simulink model "dual_single_phase_parallel_inverter_r2024a"  (R2024a)
settings: Solver=ode23t  StartTime=0.0  StopTime=0.25  MaxStep=5e-6  RelTol=1e-4
model workspace (MAT data in the model file):
  Paux1_W = 1
  Paux2_W = 1
libraries: nesl_utility x41, fl_lib x39, ee_lib x31, simulink x6
(part 1 of 4)
settings Model: Creator=chidan  LastModifiedBy=chidan

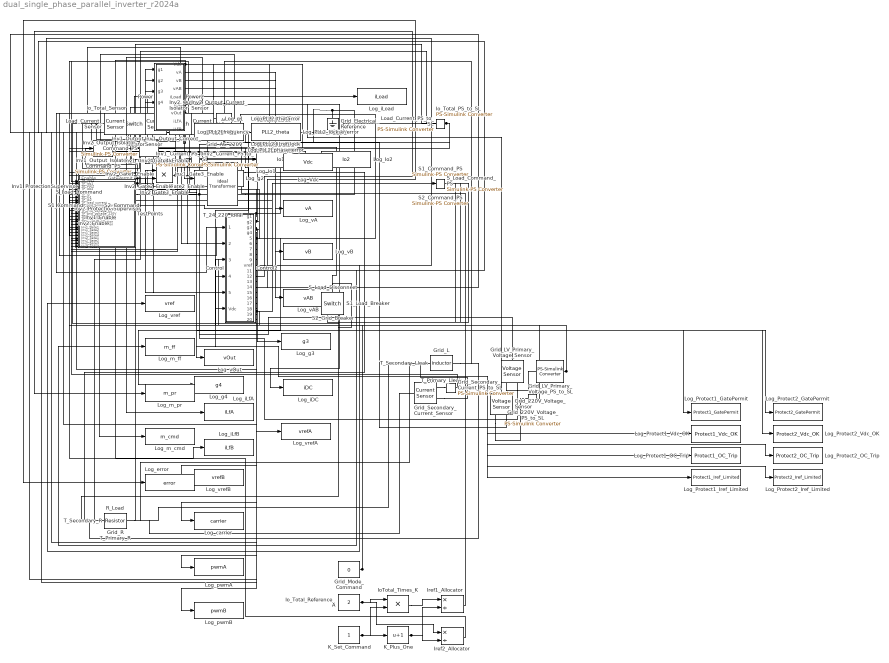
== system dual_single_phase_parallel_inverter_r2024a ==
  Control : Subsystem
  Control2 : Subsystem
  Grid_220V_Voltage_PS_to_SL : nesl_utility/PS-Simulink Converter  PhysicalDomain=network_engine_domain  SubClassName=ps_output  LeftPortType=input  RightPortType=output  PseudoPeriodic=off  Frequencies=[]  VectorFormat=inherit  Unit=inherit  AffineConversion=off
  Grid_220V_Voltage_Sensor : fl_lib/Electrical/Electrical Sensors/Voltage Sensor
  Grid_AC_220V : fl_lib/Electrical/Electrical Sources/AC Voltage Source  amp=220*sqrt(2) V  shift=0 rad  frequency=50 Hz
  Grid_Electrical_Reference : fl_lib/Electrical/Electrical Elements/Electrical Reference
  Grid_L : ee_lib/Passive/Inductor  l=1e-3 H  enable_L_tol=ee.enum.toleranceApplication.none  L_tol=20  tol_distribution=ee.enum.toleranceDistribution.uniform  nSigma=4  r=0.1 Ohm  g=1e-9 1/Ohm  enable_operating_limits=ee.enum.enable.no  operating_limit_action=ee.enum.passive.reportOpLim.warn  max_working_current=1 A  power_rating=1 W  enable_faults=ee.enum.enable.no  fault_action=simscape.enum.assert.action.none  lambdaPercent=50  k_faulted=0.9999  turnsShort=ee.enum.passive.inductor.turnsShortOption.no  openCct=ee.enum.enable.no  groundShort=ee.enum.passive.inductor.groundShortOption.no  groundShortG=0 1/Ohm  tau_fault=1e-3 s  fault_trigger=ee.enum.faults.faultTrigger.temporal  t_fault=1 s  max_permissible_voltage=100 V  n_fail_on_voltage=1  max_permissible_current=1 A  t_fail_on_current=1 s  i_L_specify=off  i_L_priority=High  i_L=0 A  i_L_nominal_specify=off  i_L_nominal_value=1  i_L_nominal_unit=A  faulted_specify=off  faulted_priority=None  faulted=0
  Grid_LV_Primary_Voltage_PS_to_SL : nesl_utility/PS-Simulink Converter  PhysicalDomain=network_engine_domain  SubClassName=ps_output  LeftPortType=input  RightPortType=output  PseudoPeriodic=off  Frequencies=[]  VectorFormat=inherit  Unit=inherit  AffineConversion=off
  Grid_LV_Primary_Voltage_Sensor : fl_lib/Electrical/Electrical Sensors/Voltage Sensor
  Grid_Mode_Command : Constant  Value=0
  Grid_R : ee_lib/Passive/Resistor  R=0.5 Ohm  enable_R_tol=ee.enum.toleranceApplication.none  R_tol=5  tol_distribution=ee.enum.toleranceDistribution.uniform  nSigma=4  enable_operating_limits=ee.enum.enable.no  operating_limit_action=ee.enum.passive.reportOpLim.warn  power_rating=1 W  max_working_voltage=100 V  enable_faults=ee.enum.enable.no  fault_action=simscape.enum.assert.action.none  R_faulted=inf Ohm  fault_trigger=ee.enum.faults.faultTrigger.temporal  t_fault=1 s  max_permissible_current=1 A  t_fail_on_current=1 s  noise_mode=ee.enum.sources.noise.Disabled  Tdevice=25 degC  sample_time=1e-3 s  repeatability=ee.enum.ic.repeatability.notRepeatable  user_seed=0  auto_seed=2348838240  faulted_specify=off  faulted_priority=None  faulted=0  power_derating_T1=70 degC  power_derating_T2=155 degC  operating_temperature_range_vec=[-50, 150] degC  alpha=3.93e-3 1/K  Tmeas=25 degC  thermal_mass=100 J/K  temperature_specify=off  temperature_priority=High  temperature=298.15 K  temperature_nominal_specify=off  temperature_nominal_value=1  temperature_nominal_unit=K
  Grid_Secondary_Current_PS_to_SL : nesl_utility/PS-Simulink Converter  PhysicalDomain=network_engine_domain  SubClassName=ps_output  LeftPortType=input  RightPortType=output  PseudoPeriodic=off  Frequencies=[]  VectorFormat=inherit  Unit=inherit  AffineConversion=off
  Grid_Secondary_Current_Sensor : fl_lib/Electrical/Electrical Sensors/Current Sensor
  Inv1_Current_PS_to_SL : nesl_utility/PS-Simulink Converter  PhysicalDomain=network_engine_domain  SubClassName=ps_output  LeftPortType=input  RightPortType=output  PseudoPeriodic=off  Frequencies=[]  VectorFormat=inherit  Unit=inherit  AffineConversion=off
  Inv1_Enable : Constant
  Inv1_Gate1_Enable : Product
  Inv1_Gate2_Enable : Product
  Inv1_Gate3_Enable : Product
  Inv1_Gate4_Enable : Product
  Inv1_Output_Current_Sensor : fl_lib/Electrical/Electrical Sensors/Current Sensor
  Inv1_Output_Isolator : fl_lib/Electrical/Electrical Elements/Switch  R_closed=0.001 Ohm  G_open=1e-8 1/Ohm  Threshold=0.5  i_specify=off  i_priority=None  i=0 A  i_nominal_specify=off  i_nominal_value=1  i_nominal_unit=A  v_specify=off  v_priority=None  v=0 V  v_nominal_specify=off  v_nominal_value=1  v_nominal_unit=V
  Inv1_Output_Isolator_Command_PS : nesl_utility/Simulink-PS Converter  PhysicalDomain=network_engine_domain  SubClassName=ps_input  LeftPortType=input  RightPortType=output  PseudoPeriodic=off  Frequencies=[]  NoiseDistribution=none  NoiseParameters=[]  Unit=1  AffineConversion=off  FilteringAndDerivatives=provide  SimscapeFilterOrder=1  InputFilterTimeConstant=0.001  UdotUserProvided=0
  Inv1_ProtectionSupervisor : Subsystem
  Inv2_Current_PS_to_SL : nesl_utility/PS-Simulink Converter  PhysicalDomain=network_engine_domain  SubClassName=ps_output  LeftPortType=input  RightPortType=output  PseudoPeriodic=off  Frequencies=[]  VectorFormat=inherit  Unit=inherit  AffineConversion=off
  Inv2_Enable : Constant
  Inv2_Gate1_Enable : Product
  Inv2_Gate2_Enable : Product
  Inv2_Gate3_Enable : Product
  Inv2_Gate4_Enable : Product
  Inv2_Output_Current_Sensor : fl_lib/Electrical/Electrical Sensors/Current Sensor
  Inv2_Output_Isolator : fl_lib/Electrical/Electrical Elements/Switch  R_closed=0.001 Ohm  G_open=1e-8 1/Ohm  Threshold=0.5  i_specify=off  i_priority=None  i=0 A  i_nominal_specify=off  i_nominal_value=1  i_nominal_unit=A  v_specify=off  v_priority=None  v=0 V  v_nominal_specify=off  v_nominal_value=1  v_nominal_unit=V
  Inv2_Output_Isolator_Command_PS : nesl_utility/Simulink-PS Converter  PhysicalDomain=network_engine_domain  SubClassName=ps_input  LeftPortType=input  RightPortType=output  PseudoPeriodic=off  Frequencies=[]  NoiseDistribution=none  NoiseParameters=[]  Unit=1  AffineConversion=off  FilteringAndDerivatives=provide  SimscapeFilterOrder=1  InputFilterTimeConstant=0.001  UdotUserProvided=0
  Inv2_ProtectionSupervisor : Subsystem
  IoTotal_Times_K : Product  Inputs=**
  Io_Total_PS_to_SL : nesl_utility/PS-Simulink Converter  PhysicalDomain=network_engine_domain  SubClassName=ps_output  LeftPortType=input  RightPortType=output  PseudoPeriodic=off  Frequencies=[]  VectorFormat=inherit  Unit=inherit  AffineConversion=off
  Io_Total_Reference_A : Constant  Value=2
  Io_Total_Sensor : fl_lib/Electrical/Electrical Sensors/Current Sensor
  Iref1_Allocator : Product  Inputs=*/
  Iref2_Allocator : Product  Inputs=*/
  K_Plus_One : Bias  Bias=1  SaturateOnIntegerOverflow=off
  K_Set_Command : Constant
  Load_Current_PS_to_SL : nesl_utility/PS-Simulink Converter  PhysicalDomain=network_engine_domain  SubClassName=ps_output  LeftPortType=input  RightPortType=output  PseudoPeriodic=off  Frequencies=[]  VectorFormat=inherit  Unit=inherit  AffineConversion=off
  Load_Current_Sensor : fl_lib/Electrical/Electrical Sensors/Current Sensor
  Log_Inv1_Gate1 : ToWorkspace  VariableName=Inv1_gate1  SaveFormat=Timeseries  SampleTime=-1
  Log_Inv1_Gate2 : ToWorkspace  VariableName=Inv1_gate2  SaveFormat=Timeseries  SampleTime=-1
  Log_Inv1_Gate3 : ToWorkspace  VariableName=Inv1_gate3  SaveFormat=Timeseries  SampleTime=-1
  Log_Inv1_Gate4 : ToWorkspace  VariableName=Inv1_gate4  SaveFormat=Timeseries  SampleTime=-1
  Log_Inv2_Ctrl_g1 : ToWorkspace  VariableName=Inv2_ctrl_g1  SaveFormat=Timeseries  SampleTime=-1
  Log_Inv2_Ctrl_g2 : ToWorkspace  VariableName=Inv2_ctrl_g2  SaveFormat=Timeseries  SampleTime=-1
  Log_Inv2_Ctrl_g3 : ToWorkspace  VariableName=Inv2_ctrl_g3  SaveFormat=Timeseries  SampleTime=-1
  Log_Inv2_Ctrl_g4 : ToWorkspace  VariableName=Inv2_ctrl_g4  SaveFormat=Timeseries  SampleTime=-1
  Log_Inv2_Gate1 : ToWorkspace  VariableName=Inv2_gate1  SaveFormat=Timeseries  SampleTime=-1
  Log_Inv2_Gate2 : ToWorkspace  VariableName=Inv2_gate2  SaveFormat=Timeseries  SampleTime=-1
  Log_Inv2_Gate3 : ToWorkspace  VariableName=Inv2_gate3  SaveFormat=Timeseries  SampleTime=-1
  Log_Inv2_Gate4 : ToWorkspace  VariableName=Inv2_gate4  SaveFormat=Timeseries  SampleTime=-1
  Log_Inv2_Vdc : ToWorkspace  VariableName=Inv2_Vdc  SaveFormat=Timeseries  SampleTime=-1
  Log_Inv2_carrier : ToWorkspace  VariableName=Inv2_carrier  SaveFormat=Timeseries  SampleTime=-1
  Log_Inv2_error : ToWorkspace  VariableName=Inv2_error  SaveFormat=Timeseries  SampleTime=-1
  Log_Inv2_iDC : ToWorkspace  VariableName=Inv2_iDC  SaveFormat=Timeseries  SampleTime=-1
  Log_Inv2_iLfA : ToWorkspace  VariableName=Inv2_iLfA  SaveFormat=Timeseries  SampleTime=-1
  Log_Inv2_iLfB : ToWorkspace  VariableName=Inv2_iLfB  SaveFormat=Timeseries  SampleTime=-1
  Log_Inv2_iLoad : ToWorkspace  VariableName=Inv2_iLoad  SaveFormat=Timeseries  SampleTime=-1
  Log_Inv2_m_cmd : ToWorkspace  VariableName=Inv2_m_cmd  SaveFormat=Timeseries  SampleTime=-1
  Log_Inv2_m_ff : ToWorkspace  VariableName=Inv2_m_ff  SaveFormat=Timeseries  SampleTime=-1
  Log_Inv2_m_pr : ToWorkspace  VariableName=Inv2_m_pr  SaveFormat=Timeseries  SampleTime=-1
  Log_Inv2_pwmA : ToWorkspace  VariableName=Inv2_pwmA  SaveFormat=Timeseries  SampleTime=-1
  Log_Inv2_pwmB : ToWorkspace  VariableName=Inv2_pwmB  SaveFormat=Timeseries  SampleTime=-1
  Log_Inv2_vA : ToWorkspace  VariableName=Inv2_vA  SaveFormat=Timeseries  SampleTime=-1
  Log_Inv2_vAB : ToWorkspace  VariableName=Inv2_vAB  SaveFormat=Timeseries  SampleTime=-1
  Log_Inv2_vB : ToWorkspace  VariableName=Inv2_vB  SaveFormat=Timeseries  SampleTime=-1
  Log_Inv2_vOut : ToWorkspace  VariableName=Inv2_vOut  SaveFormat=Timeseries  SampleTime=-1
  Log_Inv2_vref : ToWorkspace  VariableName=Inv2_vref  SaveFormat=Timeseries  SampleTime=-1
  Log_Inv2_vrefA : ToWorkspace  VariableName=Inv2_vrefA  SaveFormat=Timeseries  SampleTime=-1
  Log_Inv2_vrefB : ToWorkspace  VariableName=Inv2_vrefB  SaveFormat=Timeseries  SampleTime=-1
  Log_Io1 : ToWorkspace  VariableName=Io1  SaveFormat=Timeseries  SampleTime=-1
  Log_Io2 : ToWorkspace  VariableName=Io2  SaveFormat=Timeseries  SampleTime=-1
  Log_Io_Total : ToWorkspace  VariableName=Io_total  SaveFormat=Timeseries  SampleTime=-1
  Log_Load_Current : ToWorkspace  VariableName=I_load  SaveFormat=Timeseries  SampleTime=-1
  Log_PLL1_frequency : ToWorkspace  VariableName=PLL1_frequency_Hz  SaveFormat=Timeseries  SampleTime=-1
  Log_PLL1_i_error : ToWorkspace  VariableName=PLL1_i_error_A  SaveFormat=Timeseries  SampleTime=-1
  Log_PLL1_i_ref : ToWorkspace  VariableName=PLL1_i_ref_A  SaveFormat=Timeseries  SampleTime=-1
  Log_PLL1_lock : ToWorkspace  VariableName=PLL1_lock  SaveFormat=Timeseries  SampleTime=-1
  Log_PLL1_phase_error : ToWorkspace  VariableName=PLL1_phase_error  SaveFormat=Timeseries  SampleTime=-1
  Log_PLL1_theta : ToWorkspace  VariableName=PLL1_theta  SaveFormat=Timeseries  SampleTime=-1
  Log_PLL2_frequency : ToWorkspace  VariableName=PLL2_frequency_Hz  SaveFormat=Timeseries  SampleTime=-1
  Log_PLL2_i_error : ToWorkspace  VariableName=PLL2_i_error_A  SaveFormat=Timeseries  SampleTime=-1
  Log_PLL2_i_ref : ToWorkspace  VariableName=PLL2_i_ref_A  SaveFormat=Timeseries  SampleTime=-1
  Log_PLL2_lock : ToWorkspace  VariableName=PLL2_lock  SaveFormat=Timeseries  SampleTime=-1
  Log_PLL2_phase_error : ToWorkspace  VariableName=PLL2_phase_error  SaveFormat=Timeseries  SampleTime=-1
  Log_PLL2_theta : ToWorkspace  VariableName=PLL2_theta  SaveFormat=Timeseries  SampleTime=-1
  Log_Protect1_GatePermit : ToWorkspace  VariableName=Protect1_GatePermit  SaveFormat=Timeseries  SampleTime=-1
  Log_Protect1_Iref_Limited : ToWorkspace  VariableName=Protect1_Iref_Limited  SaveFormat=Timeseries  SampleTime=-1
  Log_Protect1_OC_Trip : ToWorkspace  VariableName=Protect1_OC_Trip  SaveFormat=Timeseries  SampleTime=-1
  Log_Protect1_Vdc_OK : ToWorkspace  VariableName=Protect1_Vdc_OK  SaveFormat=Timeseries  SampleTime=-1
  Log_Protect2_GatePermit : ToWorkspace  VariableName=Protect2_GatePermit  SaveFormat=Timeseries  SampleTime=-1
  Log_Protect2_Iref_Limited : ToWorkspace  VariableName=Protect2_Iref_Limited  SaveFormat=Timeseries  SampleTime=-1
  Log_Protect2_OC_Trip : ToWorkspace  VariableName=Protect2_OC_Trip  SaveFormat=Timeseries  SampleTime=-1
  Log_Protect2_Vdc_OK : ToWorkspace  VariableName=Protect2_Vdc_OK  SaveFormat=Timeseries  SampleTime=-1
  Log_Vdc : ToWorkspace  VariableName=Vdc  SaveFormat=Timeseries  SampleTime=-1
  Log_carrier : ToWorkspace  VariableName=carrier  SaveFormat=Timeseries  SampleTime=-1
  Log_error : ToWorkspace  VariableName=error  SaveFormat=Timeseries  SampleTime=-1
  Log_g1 : ToWorkspace  VariableName=g1  SaveFormat=Timeseries  SampleTime=-1
  Log_g2 : ToWorkspace  VariableName=g2  SaveFormat=Timeseries  SampleTime=-1
  Log_g3 : ToWorkspace  VariableName=g3  SaveFormat=Timeseries  SampleTime=-1
  Log_g4 : ToWorkspace  VariableName=g4  SaveFormat=Timeseries  SampleTime=-1
  Log_iDC : ToWorkspace  VariableName=iDC  SaveFormat=Timeseries  SampleTime=-1
  Log_iLfA : ToWorkspace  VariableName=iLfA  SaveFormat=Timeseries  SampleTime=-1
  Log_iLfB : ToWorkspace  VariableName=iLfB  SaveFormat=Timeseries  SampleTime=-1
  Log_iLoad : ToWorkspace  VariableName=iLoad  SaveFormat=Timeseries  SampleTime=-1
  Log_m_cmd : ToWorkspace  VariableName=m_cmd  SaveFormat=Timeseries  SampleTime=-1
  Log_m_ff : ToWorkspace  VariableName=m_ff  SaveFormat=Timeseries  SampleTime=-1
  Log_m_pr : ToWorkspace  VariableName=m_pr  SaveFormat=Timeseries  SampleTime=-1
  Log_pwmA : ToWorkspace  VariableName=pwmA  SaveFormat=Timeseries  SampleTime=-1
  Log_pwmB : ToWorkspace  VariableName=pwmB  SaveFormat=Timeseries  SampleTime=-1
  Log_vA : ToWorkspace  VariableName=vA  SaveFormat=Timeseries  SampleTime=-1
  Log_vAB : ToWorkspace  VariableName=vAB  SaveFormat=Timeseries  SampleTime=-1
  Log_vB : ToWorkspace  VariableName=vB  SaveFormat=Timeseries  SampleTime=-1
  Log_vOut : ToWorkspace  VariableName=vOut  SaveFormat=Timeseries  SampleTime=-1
  Log_vref : ToWorkspace  VariableName=vref  SaveFormat=Timeseries  SampleTime=-1
  Log_vrefA : ToWorkspace  VariableName=vrefA  SaveFormat=Timeseries  SampleTime=-1
  Log_vrefB : ToWorkspace  VariableName=vrefB  SaveFormat=Timeseries  SampleTime=-1
  Power : Subsystem
  Power2 : Subsystem
  R_Load : ee_lib/Passive/Resistor  R=12 Ohm  enable_R_tol=ee.enum.toleranceApplication.none  R_tol=5  tol_distribution=ee.enum.toleranceDistribution.uniform  nSigma=4  enable_operating_limits=ee.enum.enable.no  operating_limit_action=ee.enum.passive.reportOpLim.warn  power_rating=1 W  max_working_voltage=100 V  enable_faults=ee.enum.enable.no  fault_action=simscape.enum.assert.action.none  R_faulted=inf Ohm  fault_trigger=ee.enum.faults.faultTrigger.temporal  t_fault=1 s  max_permissible_current=1 A  t_fail_on_current=1 s  noise_mode=ee.enum.sources.noise.Disabled  Tdevice=25 degC  sample_time=1e-3 s  repeatability=ee.enum.ic.repeatability.notRepeatable  user_seed=0  auto_seed=3922919431  faulted_specify=off  faulted_priority=None  faulted=0  power_derating_T1=70 degC  power_derating_T2=155 degC  operating_temperature_range_vec=[-50, 150] degC  alpha=3.93e-3 1/K  Tmeas=25 degC  thermal_mass=100 J/K  temperature_specify=off  temperature_priority=High  temperature=298.15 K  temperature_nominal_specify=off  temperature_nominal_value=1  temperature_nominal_unit=K
  S1_Command : Constant
  S1_Command_PS : nesl_utility/Simulink-PS Converter  PhysicalDomain=network_engine_domain  SubClassName=ps_input  LeftPortType=input  RightPortType=output  PseudoPeriodic=off  Frequencies=[]  NoiseDistribution=none  NoiseParameters=[]  Unit=1  AffineConversion=off  FilteringAndDerivatives=provide  SimscapeFilterOrder=1  InputFilterTimeConstant=0.001  UdotUserProvided=0
  S1_Load_Breaker : fl_lib/Electrical/Electrical Elements/Switch  R_closed=0.01 Ohm  G_open=1e-8 1/Ohm  Threshold=0.5  i_specify=off  i_priority=None  i=0 A  i_nominal_specify=off  i_nominal_value=1  i_nominal_unit=A  v_specify=off  v_priority=None  v=0 V  v_nominal_specify=off  v_nominal_value=1  v_nominal_unit=V
  S2_Command : Constant  Value=0
  S2_Command_PS : nesl_utility/Simulink-PS Converter  PhysicalDomain=network_engine_domain  SubClassName=ps_input  LeftPortType=input  RightPortType=output  PseudoPeriodic=off  Frequencies=[]  NoiseDistribution=none  NoiseParameters=[]  Unit=1  AffineConversion=off  FilteringAndDerivatives=provide  SimscapeFilterOrder=1  InputFilterTimeConstant=0.001  UdotUserProvided=0
  S2_Grid_Breaker : fl_lib/Electrical/Electrical Elements/Switch  R_closed=0.01 Ohm  G_open=1e-8 1/Ohm  Threshold=0.5  i_specify=off  i_priority=None  i=0 A  i_nominal_specify=off  i_nominal_value=1  i_nominal_unit=A  v_specify=off  v_priority=None  v=0 V  v_nominal_specify=off  v_nominal_value=1  v_nominal_unit=V
  S_Load_Command : Constant
  S_Load_Command_PS : nesl_utility/Simulink-PS Converter  PhysicalDomain=network_engine_domain  SubClassName=ps_input  LeftPortType=input  RightPortType=output  PseudoPeriodic=off  Frequencies=[]  NoiseDistribution=none  NoiseParameters=[]  Unit=1  AffineConversion=off  FilteringAndDerivatives=provide  SimscapeFilterOrder=1  InputFilterTimeConstant=0.001  UdotUserProvided=0
  S_Load_Disconnect : fl_lib/Electrical/Electrical Elements/Switch  R_closed=0.01 Ohm  G_open=1e-8 1/Ohm  Threshold=0.5  i_specify=off  i_priority=None  i=0 A  i_nominal_specify=off  i_nominal_value=1  i_nominal_unit=A  v_specify=off  v_priority=None  v=0 V  v_nominal_specify=off  v_nominal_value=1  v_nominal_unit=V
  T_24_220_Ideal : fl_lib/Electrical/Electrical Elements/Ideal Transformer  n=24/220  i1_specify=off  i1_priority=None  i1=0 A  i1_nominal_specify=off  i1_nominal_value=1  i1_nominal_unit=A  v1_specify=off  v1_priority=None  v1=0 V  v1_nominal_specify=off  v1_nominal_value=1  v1_nominal_unit=V  i2_specify=off  i2_priority=None  i2=0 A  i2_nominal_specify=off  i2_nominal_value=1  i2_nominal_unit=A  v2_specify=off  v2_priority=None  v2=0 V  v2_nominal_specify=off  v2_nominal_value=1  v2_nominal_unit=V
  T_Primary_Lleak : ee_lib/Passive/Inductor  l=50e-6 H  enable_L_tol=ee.enum.toleranceApplication.none  L_tol=20  tol_distribution=ee.enum.toleranceDistribution.uniform  nSigma=4  r=0.01 Ohm  g=1e-9 1/Ohm  enable_operating_limits=ee.enum.enable.no  operating_limit_action=ee.enum.passive.reportOpLim.warn  max_working_current=1 A  power_rating=1 W  enable_faults=ee.enum.enable.no  fault_action=simscape.enum.assert.action.none  lambdaPercent=50  k_faulted=0.9999  turnsShort=ee.enum.passive.inductor.turnsShortOption.no  openCct=ee.enum.enable.no  groundShort=ee.enum.passive.inductor.groundShortOption.no  groundShortG=0 1/Ohm  tau_fault=1e-3 s  fault_trigger=ee.enum.faults.faultTrigger.temporal  t_fault=1 s  max_permissible_voltage=100 V  n_fail_on_voltage=1  max_permissible_current=1 A  t_fail_on_current=1 s  i_L_specify=off  i_L_priority=High  i_L=0 A  i_L_nominal_specify=off  i_L_nominal_value=1  i_L_nominal_unit=A  faulted_specify=off  faulted_priority=None  faulted=0
  T_Primary_R : ee_lib/Passive/Resistor  R=0.05 Ohm  enable_R_tol=ee.enum.toleranceApplication.none  R_tol=5  tol_distribution=ee.enum.toleranceDistribution.uniform  nSigma=4  enable_operating_limits=ee.enum.enable.no  operating_limit_action=ee.enum.passive.reportOpLim.warn  power_rating=1 W  max_working_voltage=100 V  enable_faults=ee.enum.enable.no  fault_action=simscape.enum.assert.action.none  R_faulted=inf Ohm  fault_trigger=ee.enum.faults.faultTrigger.temporal  t_fault=1 s  max_permissible_current=1 A  t_fail_on_current=1 s  noise_mode=ee.enum.sources.noise.Disabled  Tdevice=25 degC  sample_time=1e-3 s  repeatability=ee.enum.ic.repeatability.notRepeatable  user_seed=0  auto_seed=418932850  faulted_specify=off  faulted_priority=None  faulted=0  power_derating_T1=70 degC  power_derating_T2=155 degC  operating_temperature_range_vec=[-50, 150] degC  alpha=3.93e-3 1/K  Tmeas=25 degC  thermal_mass=100 J/K  temperature_specify=off  temperature_priority=High  temperature=298.15 K  temperature_nominal_specify=off  temperature_nominal_value=1  temperature_nominal_unit=K
  T_Secondary_Lleak : ee_lib/Passive/Inductor  l=4.2e-3 H  enable_L_tol=ee.enum.toleranceApplication.none  L_tol=20  tol_distribution=ee.enum.toleranceDistribution.uniform  nSigma=4  r=0.1 Ohm  g=1e-9 1/Ohm  enable_operating_limits=ee.enum.enable.no  operating_limit_action=ee.enum.passive.reportOpLim.warn  max_working_current=1 A  power_rating=1 W  enable_faults=ee.enum.enable.no  fault_action=simscape.enum.assert.action.none  lambdaPercent=50  k_faulted=0.9999  turnsShort=ee.enum.passive.inductor.turnsShortOption.no  openCct=ee.enum.enable.no  groundShort=ee.enum.passive.inductor.groundShortOption.no  groundShortG=0 1/Ohm  tau_fault=1e-3 s  fault_trigger=ee.enum.faults.faultTrigger.temporal  t_fault=1 s  max_permissible_voltage=100 V  n_fail_on_voltage=1  max_permissible_current=1 A  t_fail_on_current=1 s  i_L_specify=off  i_L_priority=High  i_L=0 A  i_L_nominal_specify=off  i_L_nominal_value=1  i_L_nominal_unit=A  faulted_specify=off  faulted_priority=None  faulted=0
  T_Secondary_R : ee_lib/Passive/Resistor  R=4.2 Ohm  enable_R_tol=ee.enum.toleranceApplication.none  R_tol=5  tol_distribution=ee.enum.toleranceDistribution.uniform  nSigma=4  enable_operating_limits=ee.enum.enable.no  operating_limit_action=ee.enum.passive.reportOpLim.warn  power_rating=1 W  max_working_voltage=100 V  enable_faults=ee.enum.enable.no  fault_action=simscape.enum.assert.action.none  R_faulted=inf Ohm  fault_trigger=ee.enum.faults.faultTrigger.temporal  t_fault=1 s  max_permissible_current=1 A  t_fail_on_current=1 s  noise_mode=ee.enum.sources.noise.Disabled  Tdevice=25 degC  sample_time=1e-3 s  repeatability=ee.enum.ic.repeatability.notRepeatable  user_seed=0  auto_seed=1196140742  faulted_specify=off  faulted_priority=None  faulted=0  power_derating_T1=70 degC  power_derating_T2=155 degC  operating_temperature_range_vec=[-50, 150] degC  alpha=3.93e-3 1/K  Tmeas=25 degC  thermal_mass=100 J/K  temperature_specify=off  temperature_priority=High  temperature=298.15 K  temperature_nominal_specify=off  temperature_nominal_value=1  temperature_nominal_unit=K
  TestPoints : Subsystem
  wires:
  Power/9(iLfB) -> Log_iLfB/1
  Power/8(iLfA) -> Log_iLfA/1, TestPoints/14(TP_inv1_filter_current)
  Control/14(error) -> Log_error/1
  Control/13(m_cmd) -> Log_m_cmd/1, TestPoints/16(TP_inv1_modulation)
  Control/12(m_pr) -> Log_m_pr/1
  Control/11(m_ff) -> Log_m_ff/1
  Control/10(vref) -> Log_vref/1
  Power/7(vOut) -> Log_vOut/1, Control/1(vOut), TestPoints/5(TP_Uo)
  Control/1(g1) -> Log_g1/1, Inv1_Gate1_Enable/1
  Control/2(g2) -> Log_g2/1, Inv1_Gate2_Enable/1
  Control/3(g3) -> Log_g3/1, Inv1_Gate3_Enable/1
  Control/4(g4) -> Log_g4/1, Inv1_Gate4_Enable/1
  Control/5(vrefA) -> Log_vrefA/1
  Control/6(vrefB) -> Log_vrefB/1
  Control/7(carrier) -> Log_carrier/1
  Control/8(pwmA) -> Log_pwmA/1
  Control/9(pwmB) -> Log_pwmB/1
  Power/1(Vdc) -> Log_Vdc/1, TestPoints/1(TP_Vdc1), Control/6(Vdc), Inv1_ProtectionSupervisor/2(Vdc)
  Power/2(vA) -> Log_vA/1
  Power/3(vB) -> Log_vB/1
  Power/4(vAB) -> Log_vAB/1
  Power/5(iLoad) -> Log_iLoad/1
  Power/6(iDC) -> Log_iDC/1, TestPoints/2(TP_Idc1)
  Power2/7(vOut) -> Control2/1(vOut), Log_Inv2_vOut/1
  Control2/1(g1) -> Inv2_Gate1_Enable/1, Log_Inv2_Ctrl_g1/1
  Control2/2(g2) -> Inv2_Gate2_Enable/1, Log_Inv2_Ctrl_g2/1
  Control2/3(g3) -> Inv2_Gate3_Enable/1, Log_Inv2_Ctrl_g3/1
  Control2/4(g4) -> Inv2_Gate4_Enable/1, Log_Inv2_Ctrl_g4/1
  Inv1_Enable/1 -> Inv1_ProtectionSupervisor/1(Enable)
  Inv1_Gate1_Enable/1 -> Power/1(g1), Log_Inv1_Gate1/1, TestPoints/18(Inv1_gate1)
  Inv1_Gate2_Enable/1 -> Power/2(g2), Log_Inv1_Gate2/1, TestPoints/19(Inv1_gate2)
  Inv1_Gate3_Enable/1 -> Power/3(g3), Log_Inv1_Gate3/1, TestPoints/20(Inv1_gate3)
  Inv1_Gate4_Enable/1 -> Power/4(g4), Log_Inv1_Gate4/1, TestPoints/21(Inv1_gate4)
  Inv2_Enable/1 -> Inv2_ProtectionSupervisor/1(Enable)
  Inv2_Gate1_Enable/1 -> Power2/1(g1), Log_Inv2_Gate1/1, TestPoints/22(Inv2_gate1)
  Inv2_Gate2_Enable/1 -> Power2/2(g2), Log_Inv2_Gate2/1, TestPoints/23(Inv2_gate2)
  Inv2_Gate3_Enable/1 -> Power2/3(g3), Log_Inv2_Gate3/1, TestPoints/24(Inv2_gate3)
  Inv2_Gate4_Enable/1 -> Power2/4(g4), Log_Inv2_Gate4/1, TestPoints/25(Inv2_gate4)
  S1_Command/1 -> S1_Command_PS/1
  S_Load_Command/1 -> S_Load_Command_PS/1
  S2_Command/1 -> S2_Command_PS/1
  Io_Total_PS_to_SL/1 -> Log_Io_Total/1, TestPoints/6(TP_Io), TestPoints/10(TP_grid_primary_current)
  Load_Current_PS_to_SL/1 -> Log_Load_Current/1, TestPoints/9(TP_load_current)
  Power2/1(Vdc) -> Log_Inv2_Vdc/1, TestPoints/3(TP_Vdc2), Control2/6(Vdc), Inv2_ProtectionSupervisor/2(Vdc)
  Power2/2(vA) -> Log_Inv2_vA/1
  Power2/3(vB) -> Log_Inv2_vB/1
  Power2/4(vAB) -> Log_Inv2_vAB/1
  Power2/5(iLoad) -> Log_Inv2_iLoad/1
  Power2/6(iDC) -> Log_Inv2_iDC/1, TestPoints/4(TP_Idc2)
  Power2/8(iLfA) -> Log_Inv2_iLfA/1, TestPoints/15(TP_inv2_filter_current)
  Power2/9(iLfB) -> Log_Inv2_iLfB/1
  Control2/5(vrefA) -> Log_Inv2_vrefA/1
  Control2/6(vrefB) -> Log_Inv2_vrefB/1
  Control2/7(carrier) -> Log_Inv2_carrier/1
  Control2/8(pwmA) -> Log_Inv2_pwmA/1
  Control2/9(pwmB) -> Log_Inv2_pwmB/1
  Control2/10(vref) -> Log_Inv2_vref/1
  Control2/11(m_ff) -> Log_Inv2_m_ff/1
  Control2/12(m_pr) -> Log_Inv2_m_pr/1
  Control2/13(m_cmd) -> Log_Inv2_m_cmd/1, TestPoints/17(TP_inv2_modulation)
  Control2/14(error) -> Log_Inv2_error/1
  Inv1_Current_PS_to_SL/1 -> Log_Io1/1, TestPoints/7(TP_Io1), Control/2(Io_Feedback), Inv1_ProtectionSupervisor/3(Iout)
  Inv2_Current_PS_to_SL/1 -> Log_Io2/1, TestPoints/8(TP_Io2), Control2/2(Io_Feedback), Inv2_ProtectionSupervisor/3(Iout)
  Grid_Secondary_Current_PS_to_SL/1 -> TestPoints/11(TP_grid_secondary_current)
  Grid_220V_Voltage_PS_to_SL/1 -> TestPoints/13(TP_grid_voltage_220V)
  Grid_LV_Primary_Voltage_PS_to_SL/1 -> TestPoints/12(TP_grid_voltage_LV), Control/4(Grid_Voltage), Control2/4(Grid_Voltage)
  K_Set_Command/1 -> K_Plus_One/1, IoTotal_Times_K/2
  Io_Total_Reference_A/1 -> IoTotal_Times_K/1, Iref2_Allocator/1
  IoTotal_Times_K/1 -> Iref1_Allocator/1
  K_Plus_One/1 -> Iref1_Allocator/2, Iref2_Allocator/2
  Grid_Mode_Command/1 -> Control/3(Grid_Mode), Control2/3(Grid_Mode)
  Iref1_Allocator/1 -> Inv1_ProtectionSupervisor/4(Iref)
  Iref2_Allocator/1 -> Inv2_ProtectionSupervisor/4(Iref)
  Control/15(PLL_theta) -> Log_PLL1_theta/1
  Control/16(PLL_frequency) -> Log_PLL1_frequency/1
  Control/17(PLL_lock) -> Log_PLL1_lock/1
  Control/18(Iref_instantaneous) -> Log_PLL1_i_ref/1
  Control/19(Current_Error) -> Log_PLL1_i_error/1
  Control/20(PLL_phase_error) -> Log_PLL1_phase_error/1
  Control2/15(PLL_theta) -> Log_PLL2_theta/1
  Control2/16(PLL_frequency) -> Log_PLL2_frequency/1
  Control2/17(PLL_lock) -> Log_PLL2_lock/1
  Control2/18(Iref_instantaneous) -> Log_PLL2_i_ref/1
  Control2/19(Current_Error) -> Log_PLL2_i_error/1
  Control2/20(PLL_phase_error) -> Log_PLL2_phase_error/1
  Inv1_ProtectionSupervisor/1(GatePermit) -> Inv1_Gate1_Enable/2, Inv1_Gate2_Enable/2, Inv1_Gate3_Enable/2, Inv1_Gate4_Enable/2, Inv1_Output_Isolator_Command_PS/1, Log_Protect1_GatePermit/1
  Inv1_ProtectionSupervisor/2(Iref_Limited) -> Control/5(Iref_RMS), Log_Protect1_Iref_Limited/1
  Inv1_ProtectionSupervisor/3(Vdc_OK) -> Log_Protect1_Vdc_OK/1
  Inv1_ProtectionSupervisor/4(OC_Trip) -> Log_Protect1_OC_Trip/1
  Inv2_ProtectionSupervisor/1(GatePermit) -> Inv2_Gate1_Enable/2, Inv2_Gate2_Enable/2, Inv2_Gate3_Enable/2, Inv2_Gate4_Enable/2, Inv2_Output_Isolator_Command_PS/1, Log_Protect2_GatePermit/1
  Inv2_ProtectionSupervisor/2(Iref_Limited) -> Control2/5(Iref_RMS), Log_Protect2_Iref_Limited/1
  Inv2_ProtectionSupervisor/3(Vdc_OK) -> Log_Protect2_Vdc_OK/1
  Inv2_ProtectionSupervisor/4(OC_Trip) -> Log_Protect2_OC_Trip/1
  connections:
  Power2/LConn2 -- Power/LConn2 -- R_Load/RConn1 -- T_24_220_Ideal/LConn2 -- Grid_LV_Primary_Voltage_Sensor/RConn2
  S1_Load_Breaker/LConn1 -- Io_Total_Sensor/RConn2 -- S2_Grid_Breaker/LConn1
  S1_Load_Breaker/RConn2 -- S_Load_Disconnect/LConn1
  S_Load_Disconnect/RConn2 -- Load_Current_Sensor/LConn1
  Load_Current_Sensor/RConn2 -- R_Load/LConn1
  S2_Grid_Breaker/RConn2 -- T_Primary_R/LConn1
  T_Primary_R/RConn1 -- T_Primary_Lleak/LConn1
  T_24_220_Ideal/LConn1 -- T_Primary_Lleak/RConn1 -- Grid_LV_Primary_Voltage_Sensor/LConn1
  T_24_220_Ideal/RConn1 -- T_Secondary_R/LConn1
  T_Secondary_R/RConn1 -- T_Secondary_Lleak/LConn1
  T_Secondary_Lleak/RConn1 -- Grid_R/LConn1
  Grid_AC_220V/LConn1 -- Grid_L/RConn1 -- Grid_220V_Voltage_Sensor/LConn1
  S1_Command_PS/RConn1 -- S1_Load_Breaker/RConn1
  S_Load_Command_PS/RConn1 -- S_Load_Disconnect/RConn1
  S2_Command_PS/RConn1 -- S2_Grid_Breaker/RConn1
  Io_Total_Sensor/RConn1 -- Io_Total_PS_to_SL/LConn1
  Load_Current_Sensor/RConn1 -- Load_Current_PS_to_SL/LConn1
  T_24_220_Ideal/RConn2 -- Grid_AC_220V/RConn1 -- Grid_220V_Voltage_Sensor/RConn2 -- Grid_Electrical_Reference/LConn1
  Io_Total_Sensor/LConn1 -- Inv1_Output_Current_Sensor/RConn2 -- Inv2_Output_Current_Sensor/RConn2
  Inv1_Output_Current_Sensor/RConn1 -- Inv1_Current_PS_to_SL/LConn1
  Inv2_Output_Current_Sensor/RConn1 -- Inv2_Current_PS_to_SL/LConn1
  Grid_R/RConn1 -- Grid_Secondary_Current_Sensor/LConn1
  Grid_Secondary_Current_Sensor/RConn2 -- Grid_L/LConn1
  Grid_Secondary_Current_Sensor/RConn1 -- Grid_Secondary_Current_PS_to_SL/LConn1
  Grid_220V_Voltage_Sensor/RConn1 -- Grid_220V_Voltage_PS_to_SL/LConn1
  Inv1_Output_Isolator/RConn2 -- Inv1_Output_Current_Sensor/LConn1
  Inv1_Output_Isolator_Command_PS/RConn1 -- Inv1_Output_Isolator/RConn1
  Inv2_Output_Isolator/RConn2 -- Inv2_Output_Current_Sensor/LConn1
  Inv2_Output_Isolator_Command_PS/RConn1 -- Inv2_Output_Isolator/RConn1
  Power/LConn1 -- Inv1_Output_Isolator/LConn1
  Power2/LConn1 -- Inv2_Output_Isolator/LConn1
  Grid_LV_Primary_Voltage_Sensor/RConn1 -- Grid_LV_Primary_Voltage_PS_to_SL/LConn1

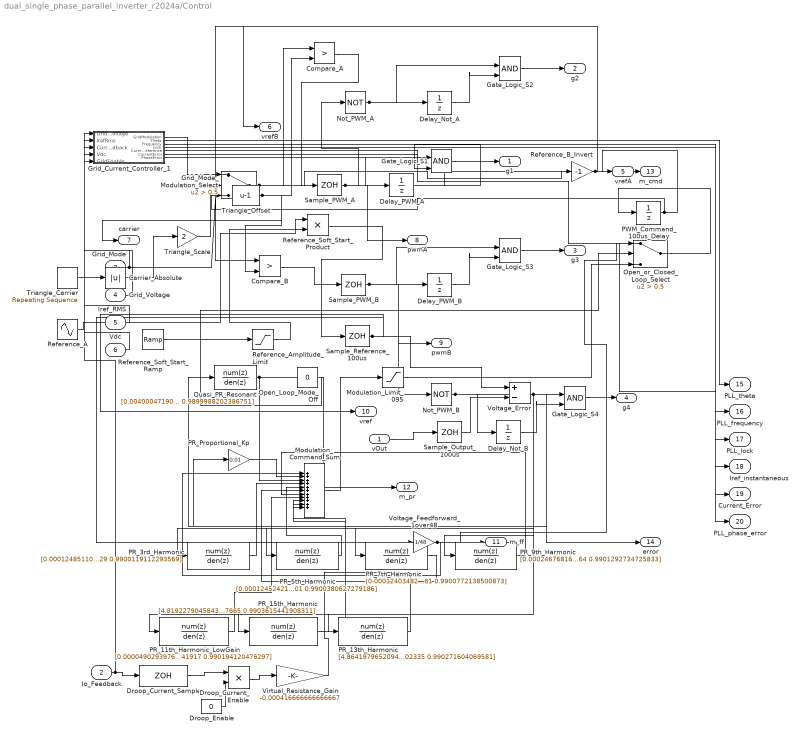
== system dual_single_phase_parallel_inverter_r2024a/Control ==
  vOut : Inport
  Io_Feedback : Inport  Port=2
  Grid_Mode : Inport  Port=3
  Grid_Voltage : Inport  Port=4
  Iref_RMS : Inport  Port=5
  Vdc : Inport  Port=6
  Carrier_Absolute : Abs  SaturateOnIntegerOverflow=off
  Compare_A : RelationalOperator  Operator=>  OutDataTypeStr=boolean  RndMeth=Simplest  InputSameDT=off
  Compare_B : RelationalOperator  Operator=>  OutDataTypeStr=boolean  RndMeth=Simplest  InputSameDT=off
  Delay_Not_A : UnitDelay  SampleTime=1e-6  HasFrameUpgradeWarning=on
  Delay_Not_B : UnitDelay  SampleTime=1e-6  HasFrameUpgradeWarning=on
  Delay_PWM_A : UnitDelay  SampleTime=1e-6  HasFrameUpgradeWarning=on
  Delay_PWM_B : UnitDelay  SampleTime=1e-6  HasFrameUpgradeWarning=on
  Droop_Current_Enable : Product
  Droop_Current_Sample : ZeroOrderHold  SampleTime=1e-4
  Droop_Enable : Constant  Value=0
  Gate_Logic_S{1..4} (4 alike) : Logic  IconShape=distinctive  AllPortsSameDT=off  OutDataTypeStr=boolean
  Grid_Current_Controller_1 : Subsystem
  Grid_Mode_Modulation_Select : Switch  Criteria=u2 > Threshold  Threshold=0.5  SaturateOnIntegerOverflow=off  InputSameDT=off
  Modulation_Command_Sum : Sum  Inputs=+++++++++++
  Modulation_Limit_095 : Saturate  UpperLimit=0.95  LowerLimit=-0.95
  Not_PWM_A : Logic  Operator=NOT  Inputs=1  IconShape=distinctive  AllPortsSameDT=off  OutDataTypeStr=boolean
  Not_PWM_B : Logic  Operator=NOT  Inputs=1  IconShape=distinctive  AllPortsSameDT=off  OutDataTypeStr=boolean
  Open_Loop_Mode_Off : Constant  Value=0
  Open_or_Closed_Loop_Select : Switch  Criteria=u2 > Threshold  Threshold=0.5  SaturateOnIntegerOverflow=off  InputSameDT=off
  PR_11th_Harmonic_LowGain : DiscreteTransferFcn  Numerator=[0.0000490293976185126 0 -0.0000490293976185126]  Denominator=[1 -1.872535374441917 0.990194120476297]  SampleTime=1e-4
  PR_13th_Harmonic : DiscreteTransferFcn  Numerator=[4.864197965209449e-05 0 -4.864197965209449e-05]  Denominator=[1 -1.826580971002335 0.990271604069581]  SampleTime=1e-4
  PR_15th_Harmonic : DiscreteTransferFcn  Numerator=[4.819227904584381e-05 0 -4.819227904584381e-05]  Denominator=[1 -1.773425121367665 0.9903615441908311]  SampleTime=1e-4
  PR_3rd_Harmonic : DiscreteTransferFcn  Numerator=[0.0001248511096330319 0 -0.0001248511096330319]  Denominator=[1 -1.981180167927029 0.9900119112293569]  SampleTime=1e-4
  PR_5th_Harmonic : DiscreteTransferFcn  Numerator=[0.00012452421590101573 0 -0.00012452421590101573]  Denominator=[1 -1.965537391896901 0.9900380627279186]  SampleTime=1e-4
  PR_7th_Harmonic : DiscreteTransferFcn  Numerator=[0.0001240348268739024 0 -0.0001240348268739024]  Denominator=[1 -1.942149710548661 0.9900772138500873]  SampleTime=1e-4
  PR_9th_Harmonic : DiscreteTransferFcn  Numerator=[0.00024676816318540615 0 -0.00024676816318540615]  Denominator=[1 -1.911108574996564 0.9901292734725833]  SampleTime=1e-4
  PR_Proportional_Kp : Gain  Gain=0.01
  PWM_Command_100us_Delay : UnitDelay  SampleTime=1e-4  HasFrameUpgradeWarning=on
  Quasi_PR_Resonant : DiscreteTransferFcn  Numerator=[0.0040004719045297 0 -0.0040004719045297]  Denominator=[1 -1.989016875948622 0.9899988202386751]  SampleTime=1e-4
  Reference_A : Sin  Amplitude=sqrt(2)*24  Frequency=2*pi*50  SampleTime=0
  Reference_Amplitude_Limit : Saturate  UpperLimit=1  LowerLimit=0
  Reference_B_Invert : Gain  Gain=-1
  Reference_Soft_Start_Product : Product
  Reference_Soft_Start_Ramp : simulink/Sources/Ramp  slope=20  start=0  InitialOutput=0
  Sample_Output_100us : ZeroOrderHold  SampleTime=1e-4
  Sample_PWM_A : ZeroOrderHold  SampleTime=1e-6
  Sample_PWM_B : ZeroOrderHold  SampleTime=1e-6
  Sample_Reference_100us : ZeroOrderHold  SampleTime=1e-4
  Triangle_Carrier : simulink/Sources/Repeating Sequence  rep_seq_t=[0 50e-6]  rep_seq_y=[-1 1]
  Triangle_Offset : Bias  Bias=-1  SaturateOnIntegerOverflow=off
  Triangle_Scale : Gain  Gain=2
  Virtual_Resistance_Gain : Gain  Gain=-0.000416666666666667
  Voltage_Error : Sum  Inputs=+-
  Voltage_Feedforward_1over48 : Gain  Gain=1/48
  g1 : Outport
  g2 : Outport  Port=2
  g3 : Outport  Port=3
  g4 : Outport  Port=4
  vrefA : Outport  Port=5
  vrefB : Outport  Port=6
  carrier : Outport  Port=7
  pwmA : Outport  Port=8
  pwmB : Outport  Port=9
  vref : Outport  Port=10
  m_ff : Outport  Port=11
  m_pr : Outport  Port=12
  m_cmd : Outport  Port=13
  error : Outport  Port=14
  PLL_theta : Outport  Port=15
  PLL_frequency : Outport  Port=16
  PLL_lock : Outport  Port=17
  Iref_instantaneous : Outport  Port=18
  Current_Error : Outport  Port=19
  PLL_phase_error : Outport  Port=20
  wires:
  Gate_Logic_S4/1 -> g4/1
  Gate_Logic_S3/1 -> g3/1
  Gate_Logic_S2/1 -> g2/1
  Gate_Logic_S1/1 -> g1/1
  Delay_Not_B/1 -> Gate_Logic_S4/2
  Delay_PWM_B/1 -> Gate_Logic_S3/2
  Delay_Not_A/1 -> Gate_Logic_S2/2
  Not_PWM_B/1 -> Gate_Logic_S4/1, Delay_Not_B/1
  Not_PWM_A/1 -> Gate_Logic_S2/1, Delay_Not_A/1
  Sample_PWM_B/1 -> pwmB/1, Gate_Logic_S3/1, Delay_PWM_B/1, Not_PWM_B/1
  Compare_B/1 -> Sample_PWM_B/1
  Triangle_Scale/1 -> Triangle_Offset/1
  Carrier_Absolute/1 -> Triangle_Scale/1
  Triangle_Carrier/1 -> Carrier_Absolute/1
  Sample_PWM_A/1 -> Not_PWM_A/1, Delay_PWM_A/1, Gate_Logic_S1/1, pwmA/1
  Delay_PWM_A/1 -> Gate_Logic_S1/2
  Modulation_Command_Sum/1 -> Modulation_Limit_095/1
  Quasi_PR_Resonant/1 -> m_pr/1, Modulation_Command_Sum/3
  PR_Proportional_Kp/1 -> Modulation_Command_Sum/2
  Voltage_Error/1 -> error/1, Quasi_PR_Resonant/1, PR_Proportional_Kp/1, PR_3rd_Harmonic/1, PR_5th_Harmonic/1, PR_7th_Harmonic/1, PR_9th_Harmonic/1, PR_11th_Harmonic_LowGain/1, PR_15th_Harmonic/1, PR_13th_Harmonic/1
  Sample_Output_100us/1 -> Voltage_Error/2
  vOut/1 -> Sample_Output_100us/1
  Sample_Reference_100us/1 -> Voltage_Error/1, Voltage_Feedforward_1over48/1, vref/1
  Reference_Amplitude_Limit/1 -> Reference_Soft_Start_Product/2
  Reference_Soft_Start_Ramp/1 -> Reference_Amplitude_Limit/1
  Reference_A/1 -> Reference_Soft_Start_Product/1
  Reference_Soft_Start_Product/1 -> Sample_Reference_100us/1
  PWM_Command_100us_Delay/1 -> vrefA/1, Grid_Mode_Modulation_Select/3
  Open_or_Closed_Loop_Select/1 -> PWM_Command_100us_Delay/1
  Reference_B_Invert/1 -> vrefB/1, Compare_B/1
  Triangle_Offset/1 -> carrier/1, Compare_B/2, Compare_A/2
  Compare_A/1 -> Sample_PWM_A/1
  Voltage_Feedforward_1over48/1 -> Modulation_Command_Sum/1, m_ff/1, Open_or_Closed_Loop_Select/1
  Open_Loop_Mode_Off/1 -> Open_or_Closed_Loop_Select/2
  Modulation_Limit_095/1 -> Open_or_Closed_Loop_Select/3
  PR_3rd_Harmonic/1 -> Modulation_Command_Sum/4
  PR_5th_Harmonic/1 -> Modulation_Command_Sum/5
  PR_7th_Harmonic/1 -> Modulation_Command_Sum/6
  PR_9th_Harmonic/1 -> Modulation_Command_Sum/7
  PR_11th_Harmonic_LowGain/1 -> Modulation_Command_Sum/8
  PR_15th_Harmonic/1 -> Modulation_Command_Sum/9
  PR_13th_Harmonic/1 -> Modulation_Command_Sum/10
  Io_Feedback/1 -> Droop_Current_Sample/1, Grid_Current_Controller_1/3(CurrentFeedback)
  Droop_Current_Sample/1 -> Droop_Current_Enable/1
  Droop_Enable/1 -> Droop_Current_Enable/2
  Droop_Current_Enable/1 -> Virtual_Resistance_Gain/1
  Virtual_Resistance_Gain/1 -> Modulation_Command_Sum/11
  Grid_Current_Controller_1/1(GridModulation) -> Grid_Mode_Modulation_Select/1
  Grid_Mode/1 -> Grid_Mode_Modulation_Select/2, Grid_Current_Controller_1/5(GridEnable)
  Grid_Mode_Modulation_Select/1 -> Compare_A/1, Reference_B_Invert/1, m_cmd/1
  Grid_Voltage/1 -> Grid_Current_Controller_1/1(GridVoltage)
  Iref_RMS/1 -> Grid_Current_Controller_1/2(IrefRms)
  Vdc/1 -> Grid_Current_Controller_1/4(Vdc)
  Grid_Current_Controller_1/2(Theta) -> PLL_theta/1
  Grid_Current_Controller_1/3(Frequency) -> PLL_frequency/1
  Grid_Current_Controller_1/4(Lock) -> PLL_lock/1
  Grid_Current_Controller_1/5(CurrentReference) -> Iref_instantaneous/1
  Grid_Current_Controller_1/6(CurrentError) -> Current_Error/1
  Grid_Current_Controller_1/7(PhaseError) -> PLL_phase_error/1

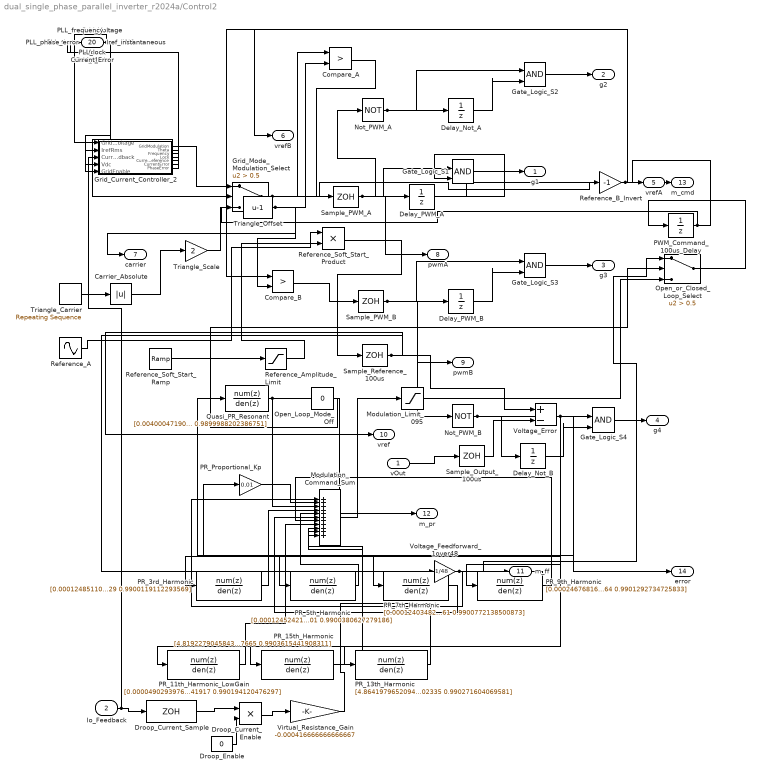
== system dual_single_phase_parallel_inverter_r2024a/Control2 ==
  vOut : Inport
  Io_Feedback : Inport  Port=2
  Grid_Mode : Inport  Port=3
  Grid_Voltage : Inport  Port=4
  Iref_RMS : Inport  Port=5
  Vdc : Inport  Port=6
  Carrier_Absolute : Abs  SaturateOnIntegerOverflow=off
  Compare_A : RelationalOperator  Operator=>  OutDataTypeStr=boolean  RndMeth=Simplest  InputSameDT=off
  Compare_B : RelationalOperator  Operator=>  OutDataTypeStr=boolean  RndMeth=Simplest  InputSameDT=off
  Delay_Not_A : UnitDelay  SampleTime=1e-6  HasFrameUpgradeWarning=on
  Delay_Not_B : UnitDelay  SampleTime=1e-6  HasFrameUpgradeWarning=on
  Delay_PWM_A : UnitDelay  SampleTime=1e-6  HasFrameUpgradeWarning=on
  Delay_PWM_B : UnitDelay  SampleTime=1e-6  HasFrameUpgradeWarning=on
  Droop_Current_Enable : Product
  Droop_Current_Sample : ZeroOrderHold  SampleTime=1e-4
  Droop_Enable : Constant  Value=0
  Gate_Logic_S{1..4} (4 alike) : Logic  IconShape=distinctive  AllPortsSameDT=off  OutDataTypeStr=boolean
  Grid_Current_Controller_2 : Subsystem
  Grid_Mode_Modulation_Select : Switch  Criteria=u2 > Threshold  Threshold=0.5  SaturateOnIntegerOverflow=off  InputSameDT=off
  Modulation_Command_Sum : Sum  Inputs=+++++++++++
  Modulation_Limit_095 : Saturate  UpperLimit=0.95  LowerLimit=-0.95
  Not_PWM_A : Logic  Operator=NOT  Inputs=1  IconShape=distinctive  AllPortsSameDT=off  OutDataTypeStr=boolean
  Not_PWM_B : Logic  Operator=NOT  Inputs=1  IconShape=distinctive  AllPortsSameDT=off  OutDataTypeStr=boolean
  Open_Loop_Mode_Off : Constant  Value=0
  Open_or_Closed_Loop_Select : Switch  Criteria=u2 > Threshold  Threshold=0.5  SaturateOnIntegerOverflow=off  InputSameDT=off
  PR_11th_Harmonic_LowGain : DiscreteTransferFcn  Numerator=[0.0000490293976185126 0 -0.0000490293976185126]  Denominator=[1 -1.872535374441917 0.990194120476297]  SampleTime=1e-4
  PR_13th_Harmonic : DiscreteTransferFcn  Numerator=[4.864197965209449e-05 0 -4.864197965209449e-05]  Denominator=[1 -1.826580971002335 0.990271604069581]  SampleTime=1e-4
  PR_15th_Harmonic : DiscreteTransferFcn  Numerator=[4.819227904584381e-05 0 -4.819227904584381e-05]  Denominator=[1 -1.773425121367665 0.9903615441908311]  SampleTime=1e-4
  PR_3rd_Harmonic : DiscreteTransferFcn  Numerator=[0.0001248511096330319 0 -0.0001248511096330319]  Denominator=[1 -1.981180167927029 0.9900119112293569]  SampleTime=1e-4
  PR_5th_Harmonic : DiscreteTransferFcn  Numerator=[0.00012452421590101573 0 -0.00012452421590101573]  Denominator=[1 -1.965537391896901 0.9900380627279186]  SampleTime=1e-4
  PR_7th_Harmonic : DiscreteTransferFcn  Numerator=[0.0001240348268739024 0 -0.0001240348268739024]  Denominator=[1 -1.942149710548661 0.9900772138500873]  SampleTime=1e-4
  PR_9th_Harmonic : DiscreteTransferFcn  Numerator=[0.00024676816318540615 0 -0.00024676816318540615]  Denominator=[1 -1.911108574996564 0.9901292734725833]  SampleTime=1e-4
  PR_Proportional_Kp : Gain  Gain=0.01
  PWM_Command_100us_Delay : UnitDelay  SampleTime=1e-4  HasFrameUpgradeWarning=on
  Quasi_PR_Resonant : DiscreteTransferFcn  Numerator=[0.0040004719045297 0 -0.0040004719045297]  Denominator=[1 -1.989016875948622 0.9899988202386751]  SampleTime=1e-4
  Reference_A : Sin  Amplitude=sqrt(2)*24  Frequency=2*pi*50  SampleTime=0
  Reference_Amplitude_Limit : Saturate  UpperLimit=1  LowerLimit=0
  Reference_B_Invert : Gain  Gain=-1
  Reference_Soft_Start_Product : Product
  Reference_Soft_Start_Ramp : simulink/Sources/Ramp  slope=20  start=0  InitialOutput=0
  Sample_Output_100us : ZeroOrderHold  SampleTime=1e-4
  Sample_PWM_A : ZeroOrderHold  SampleTime=1e-6
  Sample_PWM_B : ZeroOrderHold  SampleTime=1e-6
  Sample_Reference_100us : ZeroOrderHold  SampleTime=1e-4
  Triangle_Carrier : simulink/Sources/Repeating Sequence  rep_seq_t=[0 50e-6]  rep_seq_y=[-1 1]
  Triangle_Offset : Bias  Bias=-1  SaturateOnIntegerOverflow=off
  Triangle_Scale : Gain  Gain=2
  Virtual_Resistance_Gain : Gain  Gain=-0.000416666666666667
  Voltage_Error : Sum  Inputs=+-
  Voltage_Feedforward_1over48 : Gain  Gain=1/48
  g1 : Outport
  g2 : Outport  Port=2
  g3 : Outport  Port=3
  g4 : Outport  Port=4
  vrefA : Outport  Port=5
  vrefB : Outport  Port=6
  carrier : Outport  Port=7
  pwmA : Outport  Port=8
  pwmB : Outport  Port=9
  vref : Outport  Port=10
  m_ff : Outport  Port=11
  m_pr : Outport  Port=12
  m_cmd : Outport  Port=13
  error : Outport  Port=14
  PLL_theta : Outport  Port=15
  PLL_frequency : Outport  Port=16
  PLL_lock : Outport  Port=17
  Iref_instantaneous : Outport  Port=18
  Current_Error : Outport  Port=19
  PLL_phase_error : Outport  Port=20
  wires:
  Modulation_Limit_095/1 -> Open_or_Closed_Loop_Select/3
  Open_Loop_Mode_Off/1 -> Open_or_Closed_Loop_Select/2
  Voltage_Feedforward_1over48/1 -> Open_or_Closed_Loop_Select/1, m_ff/1, Modulation_Command_Sum/1
  Compare_A/1 -> Sample_PWM_A/1
  Triangle_Offset/1 -> Compare_A/2, Compare_B/2, carrier/1
  Reference_B_Invert/1 -> Compare_B/1, vrefB/1
  Open_or_Closed_Loop_Select/1 -> PWM_Command_100us_Delay/1
  PWM_Command_100us_Delay/1 -> vrefA/1, Grid_Mode_Modulation_Select/3
  Reference_Soft_Start_Product/1 -> Sample_Reference_100us/1
  Reference_A/1 -> Reference_Soft_Start_Product/1
  Reference_Soft_Start_Ramp/1 -> Reference_Amplitude_Limit/1
  Reference_Amplitude_Limit/1 -> Reference_Soft_Start_Product/2
  Sample_Reference_100us/1 -> vref/1, Voltage_Feedforward_1over48/1, Voltage_Error/1
  vOut/1 -> Sample_Output_100us/1
  Sample_Output_100us/1 -> Voltage_Error/2
  Voltage_Error/1 -> PR_Proportional_Kp/1, Quasi_PR_Resonant/1, error/1, PR_3rd_Harmonic/1, PR_5th_Harmonic/1, PR_7th_Harmonic/1, PR_9th_Harmonic/1, PR_11th_Harmonic_LowGain/1, PR_15th_Harmonic/1, PR_13th_Harmonic/1
  PR_Proportional_Kp/1 -> Modulation_Command_Sum/2
  Quasi_PR_Resonant/1 -> Modulation_Command_Sum/3, m_pr/1
  Modulation_Command_Sum/1 -> Modulation_Limit_095/1
  Delay_PWM_A/1 -> Gate_Logic_S1/2
  Sample_PWM_A/1 -> pwmA/1, Gate_Logic_S1/1, Delay_PWM_A/1, Not_PWM_A/1
  Triangle_Carrier/1 -> Carrier_Absolute/1
  Carrier_Absolute/1 -> Triangle_Scale/1
  Triangle_Scale/1 -> Triangle_Offset/1
  Compare_B/1 -> Sample_PWM_B/1
  Sample_PWM_B/1 -> Not_PWM_B/1, Delay_PWM_B/1, Gate_Logic_S3/1, pwmB/1
  Not_PWM_A/1 -> Delay_Not_A/1, Gate_Logic_S2/1
  Not_PWM_B/1 -> Delay_Not_B/1, Gate_Logic_S4/1
  Delay_Not_A/1 -> Gate_Logic_S2/2
  Delay_PWM_B/1 -> Gate_Logic_S3/2
  Delay_Not_B/1 -> Gate_Logic_S4/2
  Gate_Logic_S1/1 -> g1/1
  Gate_Logic_S2/1 -> g2/1
  Gate_Logic_S3/1 -> g3/1
  Gate_Logic_S4/1 -> g4/1
  PR_3rd_Harmonic/1 -> Modulation_Command_Sum/4
  PR_5th_Harmonic/1 -> Modulation_Command_Sum/5
  PR_7th_Harmonic/1 -> Modulation_Command_Sum/6
  PR_9th_Harmonic/1 -> Modulation_Command_Sum/7
  PR_11th_Harmonic_LowGain/1 -> Modulation_Command_Sum/8
  PR_15th_Harmonic/1 -> Modulation_Command_Sum/9
  PR_13th_Harmonic/1 -> Modulation_Command_Sum/10
  Io_Feedback/1 -> Droop_Current_Sample/1, Grid_Current_Controller_2/3(CurrentFeedback)
  Droop_Current_Sample/1 -> Droop_Current_Enable/1
  Droop_Enable/1 -> Droop_Current_Enable/2
  Droop_Current_Enable/1 -> Virtual_Resistance_Gain/1
  Virtual_Resistance_Gain/1 -> Modulation_Command_Sum/11
  Grid_Current_Controller_2/1(GridModulation) -> Grid_Mode_Modulation_Select/1
  Grid_Mode/1 -> Grid_Mode_Modulation_Select/2, Grid_Current_Controller_2/5(GridEnable)
  Grid_Mode_Modulation_Select/1 -> Compare_A/1, Reference_B_Invert/1, m_cmd/1
  Grid_Voltage/1 -> Grid_Current_Controller_2/1(GridVoltage)
  Iref_RMS/1 -> Grid_Current_Controller_2/2(IrefRms)
  Vdc/1 -> Grid_Current_Controller_2/4(Vdc)
  Grid_Current_Controller_2/2(Theta) -> PLL_theta/1
  Grid_Current_Controller_2/3(Frequency) -> PLL_frequency/1
  Grid_Current_Controller_2/4(Lock) -> PLL_lock/1
  Grid_Current_Controller_2/5(CurrentReference) -> Iref_instantaneous/1
  Grid_Current_Controller_2/6(CurrentError) -> Current_Error/1
  Grid_Current_Controller_2/7(PhaseError) -> PLL_phase_error/1

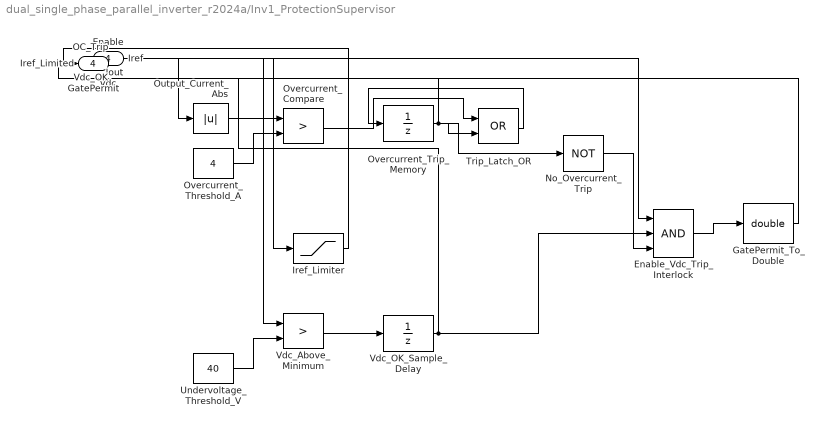
== system dual_single_phase_parallel_inverter_r2024a/Inv1_ProtectionSupervisor ==
  Enable : Inport
  Vdc : Inport  Port=2
  Iout : Inport  Port=3
  Iref : Inport  Port=4
  Enable_Vdc_Trip_Interlock : Logic  Inputs=3  AllPortsSameDT=off  OutDataTypeStr=boolean
  GatePermit_To_Double : DataTypeConversion  OutDataTypeStr=double  SaturateOnIntegerOverflow=off  RndMeth=Floor
  Iref_Limiter : Saturate  UpperLimit=2  LowerLimit=0
  No_Overcurrent_Trip : Logic  Operator=NOT  Inputs=1  AllPortsSameDT=off  OutDataTypeStr=boolean
  Output_Current_Abs : Abs  SaturateOnIntegerOverflow=off
  Overcurrent_Compare : RelationalOperator  Operator=>  OutDataTypeStr=boolean  RndMeth=Simplest  InputSameDT=off
  Overcurrent_Threshold_A : Constant  Value=4
  Overcurrent_Trip_Memory : UnitDelay  SampleTime=1e-5  HasFrameUpgradeWarning=on
  Trip_Latch_OR : Logic  Operator=OR  AllPortsSameDT=off  OutDataTypeStr=boolean
  Undervoltage_Threshold_V : Constant  Value=40
  Vdc_Above_Minimum : RelationalOperator  Operator=>  OutDataTypeStr=boolean  RndMeth=Simplest  InputSameDT=off
  Vdc_OK_Sample_Delay : UnitDelay  SampleTime=1e-5  HasFrameUpgradeWarning=on
  GatePermit : Outport
  Iref_Limited : Outport  Port=2
  Vdc_OK : Outport  Port=3
  OC_Trip : Outport  Port=4
  wires:
  Iref/1 -> Iref_Limiter/1
  Iref_Limiter/1 -> Iref_Limited/1
  Iout/1 -> Output_Current_Abs/1
  Output_Current_Abs/1 -> Overcurrent_Compare/1
  Overcurrent_Threshold_A/1 -> Overcurrent_Compare/2
  Overcurrent_Compare/1 -> Trip_Latch_OR/1
  Overcurrent_Trip_Memory/1 -> Trip_Latch_OR/2, OC_Trip/1, No_Overcurrent_Trip/1
  Trip_Latch_OR/1 -> Overcurrent_Trip_Memory/1
  Vdc/1 -> Vdc_Above_Minimum/1
  Undervoltage_Threshold_V/1 -> Vdc_Above_Minimum/2
  Vdc_Above_Minimum/1 -> Vdc_OK_Sample_Delay/1
  Enable/1 -> Enable_Vdc_Trip_Interlock/1
  No_Overcurrent_Trip/1 -> Enable_Vdc_Trip_Interlock/3
  Enable_Vdc_Trip_Interlock/1 -> GatePermit_To_Double/1
  GatePermit_To_Double/1 -> GatePermit/1
  Vdc_OK_Sample_Delay/1 -> Vdc_OK/1, Enable_Vdc_Trip_Interlock/2

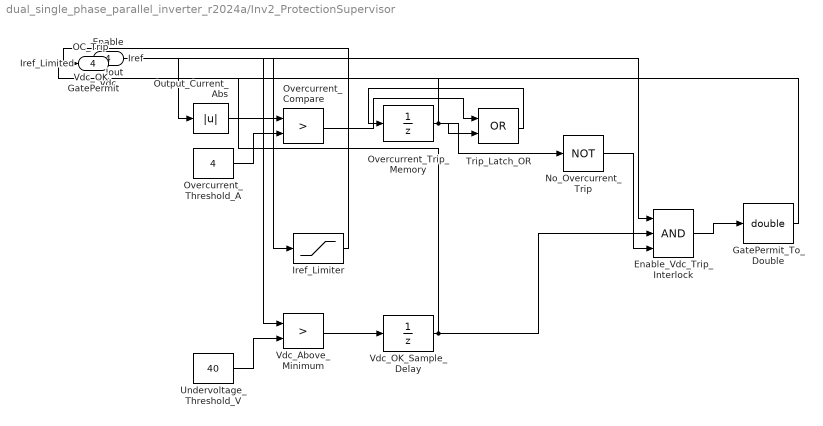
== system dual_single_phase_parallel_inverter_r2024a/Inv2_ProtectionSupervisor ==
  Enable : Inport
  Vdc : Inport  Port=2
  Iout : Inport  Port=3
  Iref : Inport  Port=4
  Enable_Vdc_Trip_Interlock : Logic  Inputs=3  AllPortsSameDT=off  OutDataTypeStr=boolean
  GatePermit_To_Double : DataTypeConversion  OutDataTypeStr=double  SaturateOnIntegerOverflow=off  RndMeth=Floor
  Iref_Limiter : Saturate  UpperLimit=2  LowerLimit=0
  No_Overcurrent_Trip : Logic  Operator=NOT  Inputs=1  AllPortsSameDT=off  OutDataTypeStr=boolean
  Output_Current_Abs : Abs  SaturateOnIntegerOverflow=off
  Overcurrent_Compare : RelationalOperator  Operator=>  OutDataTypeStr=boolean  RndMeth=Simplest  InputSameDT=off
  Overcurrent_Threshold_A : Constant  Value=4
  Overcurrent_Trip_Memory : UnitDelay  SampleTime=1e-5  HasFrameUpgradeWarning=on
  Trip_Latch_OR : Logic  Operator=OR  AllPortsSameDT=off  OutDataTypeStr=boolean
  Undervoltage_Threshold_V : Constant  Value=40
  Vdc_Above_Minimum : RelationalOperator  Operator=>  OutDataTypeStr=boolean  RndMeth=Simplest  InputSameDT=off
  Vdc_OK_Sample_Delay : UnitDelay  SampleTime=1e-5  HasFrameUpgradeWarning=on
  GatePermit : Outport
  Iref_Limited : Outport  Port=2
  Vdc_OK : Outport  Port=3
  OC_Trip : Outport  Port=4
  wires:
  Iref/1 -> Iref_Limiter/1
  Iref_Limiter/1 -> Iref_Limited/1
  Iout/1 -> Output_Current_Abs/1
  Output_Current_Abs/1 -> Overcurrent_Compare/1
  Overcurrent_Threshold_A/1 -> Overcurrent_Compare/2
  Overcurrent_Compare/1 -> Trip_Latch_OR/1
  Overcurrent_Trip_Memory/1 -> Trip_Latch_OR/2, OC_Trip/1, No_Overcurrent_Trip/1
  Trip_Latch_OR/1 -> Overcurrent_Trip_Memory/1
  Vdc/1 -> Vdc_Above_Minimum/1
  Undervoltage_Threshold_V/1 -> Vdc_Above_Minimum/2
  Vdc_Above_Minimum/1 -> Vdc_OK_Sample_Delay/1
  Enable/1 -> Enable_Vdc_Trip_Interlock/1
  No_Overcurrent_Trip/1 -> Enable_Vdc_Trip_Interlock/3
  Enable_Vdc_Trip_Interlock/1 -> GatePermit_To_Double/1
  GatePermit_To_Double/1 -> GatePermit/1
  Vdc_OK_Sample_Delay/1 -> Vdc_OK/1, Enable_Vdc_Trip_Interlock/2
